simulink model "tuning_attitudeController"  (R2022a)
settings: Solver=VariableStepAuto  StartTime=0.0  StopTime=10.0  RelTol=1e-3
values from neighbouring files (symbols this model uses):
  J = cat(2, [0 0 0]', J)    [LQRCalcs.m]    (also in init_parameters.m = diag([0.082, 0.0845, 0.1377]); main.m = diag([0.082, 0.0845, 0.1377]); parameters_buildingSimulink.m = diag([0.082, 0.0845, 0.1377]); parameters_init.m = diag([0.082, 0.0845, 0.1377]))
undefined symbols (not defined in the file or in its folder): Gain
settings Model: Creator=willg  LastModifiedBy=willg

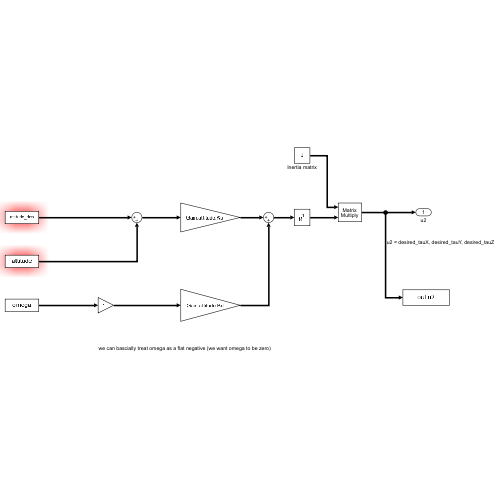
[thumbnail: Simulink's stored preview of the top-level diagram]
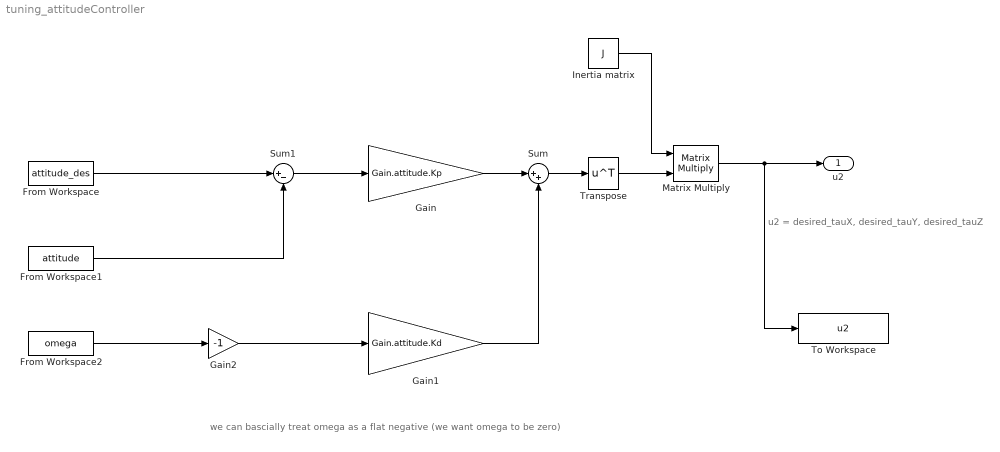
== system tuning_attitudeController ==
  note: u2 = desired_tauX, desired_tauY, desired_tauZ
  note: we can bascially treat omega as a flat negative (we want omega to be zero)
  From Workspace : FromWorkspace  VariableName=attitude_des
  From Workspace1 : FromWorkspace  VariableName=attitude
  From Workspace2 : FromWorkspace  VariableName=omega
  Gain : Gain  Gain=Gain.attitude.Kp
  Gain1 : Gain  Gain=Gain.attitude.Kd
  Gain2 : Gain  Gain=-1
  Inertia matrix : Constant  Value=J
  Matrix Multiply : Product  Multiplication=Matrix(*)
  Sum : Sum  Inputs=|++
  Sum1 : Sum  Inputs=|+-
  To Workspace : ToWorkspace  VariableName=u2  SaveFormat=Timeseries  SampleTime=-1
  Transpose : Math  Operator=transpose
  u2 : Outport
  wires:
  Gain/1 -> Sum/1
  Matrix Multiply/1 -> To Workspace/1, u2/1
  Sum/1 -> Transpose/1
  From Workspace1/1 -> Sum1/2
  Inertia matrix/1 -> Matrix Multiply/1
  Transpose/1 -> Matrix Multiply/2
  Sum1/1 -> Gain/1
  Gain1/1 -> Sum/2
  From Workspace/1 -> Sum1/1
  Gain2/1 -> Gain1/1
  From Workspace2/1 -> Gain2/1
